simulink model "control_model_new_2018a_latest"  (R2018b)
settings: Solver=VariableStepAuto  StartTime=0.0  StopTime=50  RelTol=1e-04
libraries: simulink x2
settings Model: Creator=geraldlow  LastModifiedBy=geraldlow

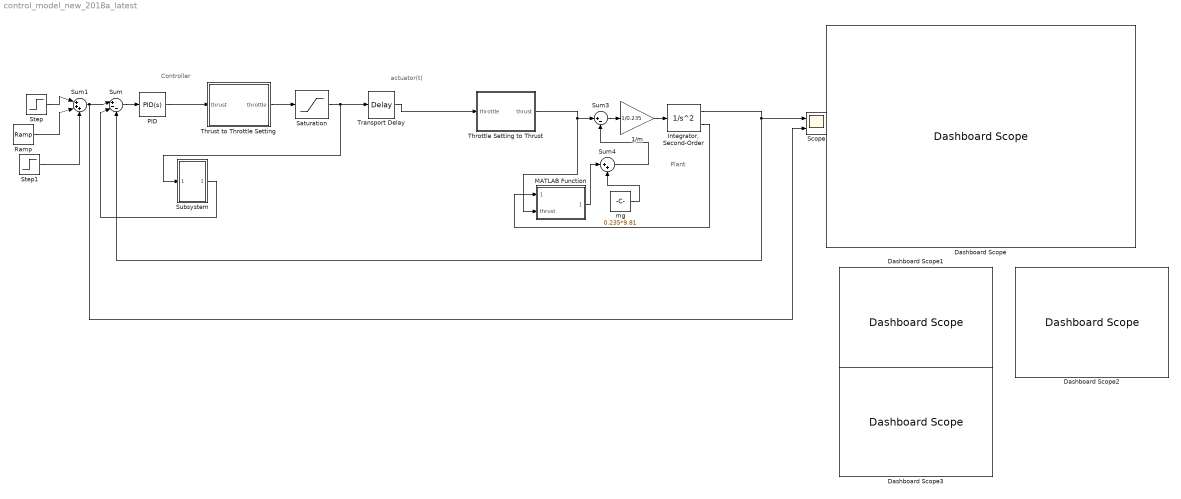
== system control_model_new_2018a_latest ==
  note: Controller
  note: Plant
  note: actuator(t)
  1/m : Gain  Gain=1/0.235
  Dashboard Scope : DashboardScope  WebBlockId=142
  Dashboard Scope1 : DashboardScope  WebBlockId=141
  Dashboard Scope2 : DashboardScope  WebBlockId=140
  Dashboard Scope3 : DashboardScope  WebBlockId=149
  "Integrator, Second-Order" : SecondOrderIntegrator  LimitX=on  LowerLimitX=0
  MATLAB Function : MATLAB Function  TreatAsAtomicUnit=on
  PID : simulink/Continuous/PID Controller  Controller=PID  Form=Parallel  TimeDomain=Continuous-time  SampleTime=-1  IntegratorMethod=Forward Euler  FilterMethod=Forward Euler  ControllerParametersSource=internal  P=1.94  I=1.57e-04  D=2.69  UseFilter=on  N=100  TunerSelectOption=Transfer Function Based (PID Tuner App)  InitialConditionSource=internal  InitialConditionForIntegrator=0  InitialConditionForFilter=0  DifferentiatorICPrevScaledInput=0  ExternalReset=none  TrackingMode=off  Kt=1  LimitOutput=off  UpperSaturationLimit=inf  LowerSaturationLimit=-inf  LinearizeAsGain=on  AntiWindupMode=none  Kb=1  POutMin=[]  POutMax=[]  IOutMin=[]  IOutMax=[]  DOutMin=[]  DOutMax=[]  NOutMin=[]  NOutMax=[]  SumOutMin=[]  SumOutMax=[]  SaturationOutMin=[]  SaturationOutMax=[]  PParamMin=[]  PParamMax=[]  IParamMin=[]  IParamMax=[]  DParamMin=[]  DParamMax=[]  NParamMin=[]  NParamMax=[]  KbParamMin=[]  KbParamMax=[]  KtParamMin=[]  KtParamMax=[]  KbOutMin=[]  KbOutMax=[]  KtOutMin=[]  KtOutMax=[]  IntegratorOutMin=[]  IntegratorOutMax=[]  FilterOutMin=[]  FilterOutMax=[]  SumI1OutMin=[]  SumI1OutMax=[]  SumI2OutMin=[]  SumI2OutMax=[]  SumI3OutMin=[]  SumI3OutMax=[]  SumI4OutMin=[]  SumI4OutMax=[]  SumDOutMin=[]  SumDOutMax=[]  DifferentiatorOutMin=[]  DifferentiatorOutMax=[]  FilterDiffOutCoefMin=[]  FilterDiffOutCoefMax=[]  ReciprocalOutMin=[]  ReciprocalOutMax=[]  SumDenOutMin=[]  SumDenOutMax=[]  SumNumOutMin=[]  SumNumOutMax=[]  DivideOutMin=[]  DivideOutMax=[]  IntegratorContinuousStateAttributes=''  IntegratorStateMustResolveToSignalObject=off  IntegratorRTWStateStorageClass=Auto  FilterContinuousStateAttributes=''  FilterStateMustResolveToSignalObject=off  FilterRTWStateStorageClass=Auto  ParallelPVariant=InternalParameters  IdealPVariant=Disabled  IVariant=InternalParameters  DVariant=InternalParameters  IntegratorVariant=Continuous  SatVariant=Disabled  AWVariant=Passthrough  PCopyVariant=Disabled  TRVariant=Disabled  FdbkBlocksVariant=Forward  IdealPFdbkVariant=Disabled  SatFdbkVariant=Disabled  DerivativeFilterVariant=ContFilter  NVariant=InternalParameters  NCopyVariant=Disabled  FilterICVariant=InternalICsFilter  IntegratorICVariant=InternalICs  ExternalResetVariant=Disabled  TRSumVariant=Passthrough  SumFdbkVariant=Disabled  SumVariant=Sum_PID
  Ramp : simulink/Sources/Ramp  slope=-.25  start=40  InitialOutput=0
  Saturation : Saturate  UpperLimit=100  LowerLimit=0
  Scope : Scope  NumInputPorts=2
  Step : Step  Time=10  SampleTime=0
  Step1 : Step  Time=20  After=.5  SampleTime=0
  Subsystem : Subsystem
  Sum : Sum  Inputs=|+--
  Sum1 : Sum  Inputs=|+++
  Sum3 : Sum  Inputs=|+-
  Sum4 : Sum  Inputs=|++
  Throttle Setting to Thrust : MATLAB Function  TreatAsAtomicUnit=on
  Thrust to Throttle Setting : MATLAB Function  TreatAsAtomicUnit=on
  Transport Delay : TransportDelay  DelayTime=.8
  mg : Constant  Value=0.235*9.81
  wires:
  Thrust to Throttle Setting/1(throttle) -> Saturation/1
  mg/1 -> Sum4/2
  Sum3/1 -> 1/m/1
  Sum1/1 -> Sum/1, Scope/2
  Sum4/1 -> Sum3/2
  MATLAB Function/1(friction) -> Sum4/1
  Throttle Setting to Thrust/1(thrust) -> Sum3/1, MATLAB Function/2(thrust)
  PID/1 -> Thrust to Throttle Setting/1(thrust)
  Saturation/1 -> Subsystem/1(In1), Transport Delay/1
  Ramp/1 -> Sum1/2
  Step1/1 -> Sum1/3
  Sum/1 -> PID/1
  Step/1 -> Sum1/1
  "Integrator, Second-Order"/1 -> Sum/3, Scope/1
  Transport Delay/1 -> Throttle Setting to Thrust/1(throttle)
  Subsystem/1(Out1) -> Sum/2
  1/m/1 -> "Integrator, Second-Order"/1
  "Integrator, Second-Order"/2 -> MATLAB Function/1(velocity)

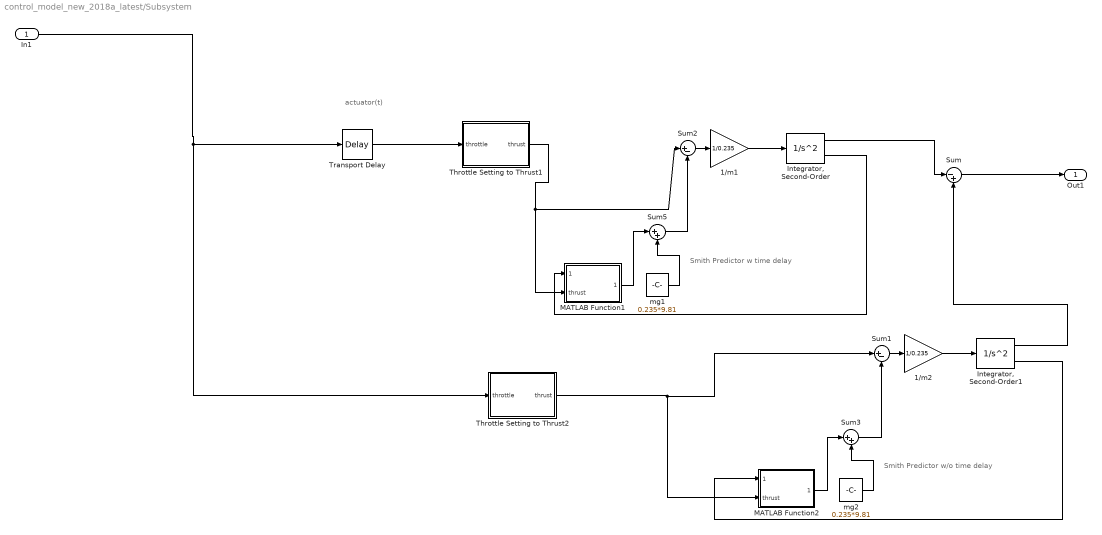
== system control_model_new_2018a_latest/Subsystem ==
  note: Smith Predictor w time delay
  note: actuator(t)
  note: Smith Predictor w/o time delay
  In1 : Inport
  1/m1 : Gain  Gain=1/0.235
  1/m2 : Gain  Gain=1/0.235
  "Integrator, Second-Order" : SecondOrderIntegrator  LimitX=on  LowerLimitX=0
  "Integrator, Second-Order1" : SecondOrderIntegrator  LimitX=on  LowerLimitX=0
  MATLAB Function1 : MATLAB Function  TreatAsAtomicUnit=on
  MATLAB Function2 : MATLAB Function  TreatAsAtomicUnit=on
  Sum : Sum  Inputs=|-+
  Sum1 : Sum  Inputs=|+-
  Sum2 : Sum  Inputs=|+-
  Sum3 : Sum  Inputs=|++
  Sum5 : Sum  Inputs=|++
  Throttle Setting to Thrust1 : MATLAB Function  TreatAsAtomicUnit=on
  Throttle Setting to Thrust2 : MATLAB Function  TreatAsAtomicUnit=on
  Transport Delay : TransportDelay  DelayTime=.8
  mg1 : Constant  Value=0.235*9.81
  mg2 : Constant  Value=0.235*9.81
  Out1 : Outport
  wires:
  1/m1/1 -> "Integrator, Second-Order"/1
  Sum2/1 -> 1/m1/1
  MATLAB Function1/1(friction) -> Sum5/1
  mg1/1 -> Sum5/2
  Throttle Setting to Thrust1/1(thrust) -> MATLAB Function1/2(thrust), Sum2/1
  Sum5/1 -> Sum2/2
  "Integrator, Second-Order"/1 -> Sum/1
  "Integrator, Second-Order1"/1 -> Sum/2
  mg2/1 -> Sum3/2
  MATLAB Function2/1(friction) -> Sum3/1
  Sum3/1 -> Sum1/2
  Sum1/1 -> 1/m2/1
  1/m2/1 -> "Integrator, Second-Order1"/1
  Sum/1 -> Out1/1
  Transport Delay/1 -> Throttle Setting to Thrust1/1(throttle)
  Throttle Setting to Thrust2/1(thrust) -> Sum1/1, MATLAB Function2/2(thrust)
  "Integrator, Second-Order"/2 -> MATLAB Function1/1(velocity)
  "Integrator, Second-Order1"/2 -> MATLAB Function2/1(velocity)
  In1/1 -> Throttle Setting to Thrust2/1(throttle), Transport Delay/1

== matlab function control_model_new_2018a_latest/Throttle Setting to Thrust ==
  data: throttle input; thrust output
function thrust = fcn(throttle)
if throttle < 1
    thrust = 0;
elseif throttle > 88
    thrust=2*9.81*.66;
else
    thrust=2*9.81*(0.1+(.66-0.1)/(88-1)*(throttle-1));
end
end

== matlab function control_model_new_2018a_latest/Thrust to Throttle Setting ==
  data: thrust input; throttle output
function throttle = fcn(thrust)
% (.66-0.1)/(88-1)*2*9.81 = 0.1263
epsilon = 0.001;
if thrust < epsilon
    throttle = 0;
else
    throttle = (thrust / 0.1263)+.8;
end
end

== matlab function control_model_new_2018a_latest/MATLAB Function ==
  data: velocity input; friction output; thrust input
function friction   = fcn(velocity, thrust)
epsilon = 0.005; %small perturbation
mg = 0.235*9.81;
% Get reasonable values for x1, x2, l
x1 = 0.0125;
x2 = 0.0125;
l = 0.221;
netforce = thrust-mg; %mg should be a constant defined.
mu = 0.15; %coeff of dynamic friction
%static friction
if abs(velocity) < epsilon && abs(netforce) < 0.13*9.81 && netforce > 0
    friction = netforce;
elseif abs(velocity) < epsilon && abs(netforce) < 0.13*9.81 && netforce < 0
    friction = -netforce;
elseif velocity > 0
    friction=2*mu*(mg*x1-thrust*x2)/l;
elseif velocity < 0
    friction=-2*mu*(mg*x1-thrust*x2)/l;
else
    friction=0;
end

== matlab function control_model_new_2018a_latest/Subsystem/MATLAB Function1 ==
  data: velocity input; friction output; thrust input
function friction   = fcn(velocity, thrust)
epsilon = 0.005; %small perturbation
mg = 0.235*9.81;
% Get reasonable values for x1, x2, l
x1 = 0.0125;
x2 = 0.0125;
l = 0.221;
netforce = thrust-mg; %mg should be a constant defined.
mu = 0.15; %coeff of dynamic friction
%static friction
if abs(velocity) < epsilon && abs(netforce) < 0.13*9.81 && netforce > 0
    friction = netforce;
elseif abs(velocity) < epsilon && abs(netforce) < 0.13*9.81 && netforce < 0
    friction = -netforce;
elseif velocity > 0
    friction=2*mu*(mg*x1-thrust*x2)/l;
elseif velocity < 0
    friction=-2*mu*(mg*x1-thrust*x2)/l;
else
    friction=0;
end

== matlab function control_model_new_2018a_latest/Subsystem/Throttle Setting to Thrust1 ==
  data: throttle input; thrust output
function thrust = fcn(throttle)
if throttle < 1
    thrust = 0;
elseif throttle > 88
    thrust=2*9.81*.66;
else
    thrust=2*9.81*(0.1+(.66-0.1)/(88-1)*(throttle-1));
end
end

== matlab function control_model_new_2018a_latest/Subsystem/Throttle Setting to Thrust2 ==
  data: throttle input; thrust output
function thrust = fcn(throttle)
if throttle < 1
    thrust = 0;
elseif throttle > 88
    thrust=2*9.81*.66;
else
    thrust=2*9.81*(0.1+(.66-0.1)/(88-1)*(throttle-1));
end
end

== matlab function control_model_new_2018a_latest/Subsystem/MATLAB Function2 ==
  data: velocity input; friction output; thrust input
function friction   = fcn(velocity, thrust)
epsilon = 0.005; %small perturbation
mg = 0.235*9.81;
% Get reasonable values for x1, x2, l
x1 = 0.0125;
x2 = 0.0125;
l = 0.221;
netforce = thrust-mg; %mg should be a constant defined.
mu = 0.15; %coeff of dynamic friction
%static friction
if abs(velocity) < epsilon && abs(netforce) < 0.13*9.81 && netforce > 0
    friction = netforce;
elseif abs(velocity) < epsilon && abs(netforce) < 0.13*9.81 && netforce < 0
    friction = -netforce;
elseif velocity > 0
    friction=2*mu*(mg*x1-thrust*x2)/l;
elseif velocity < 0
    friction=-2*mu*(mg*x1-thrust*x2)/l;
else
    friction=0;
end
